simulink model "Assignment5"  (R2014a)
settings: Solver=FixedStepDiscrete  StartTime=0.0  StopTime=10.0  FixedStep=1  RelTol=1e-3
libraries: hdlsllib x19, simulink x6
settings Model: Creator=ramirezlara.h  LastModifiedBy=vu.du

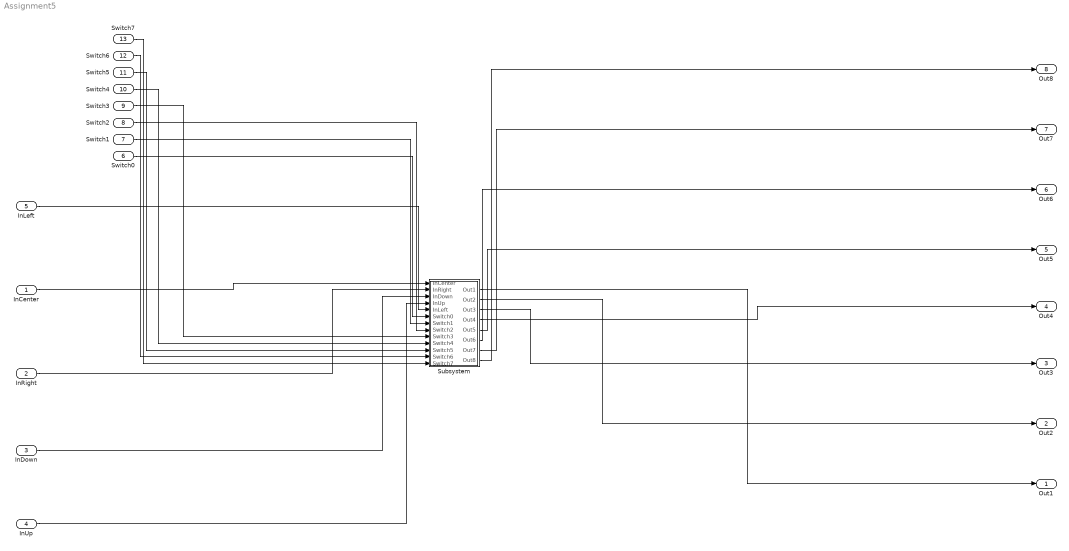
== system Assignment5 ==
  InCenter : Inport
  InRight : Inport  Port=2
  InDown : Inport  Port=3
  InUp : Inport  Port=4
  InLeft : Inport  Port=5
  Switch0 : Inport  Port=6  OutDataTypeStr=boolean
  Switch1 : Inport  Port=7  OutDataTypeStr=boolean
  Switch2 : Inport  Port=8  OutDataTypeStr=boolean
  Switch3 : Inport  Port=9  OutDataTypeStr=boolean
  Switch4 : Inport  Port=10  OutDataTypeStr=boolean
  Switch5 : Inport  Port=11  OutDataTypeStr=boolean
  Switch6 : Inport  Port=12  OutDataTypeStr=boolean
  Switch7 : Inport  Port=13  OutDataTypeStr=boolean
  Subsystem : Subsystem  TreatAsAtomicUnit=on
  Out1 : Outport
  Out2 : Outport  Port=2
  Out3 : Outport  Port=3
  Out4 : Outport  Port=4
  Out5 : Outport  Port=5
  Out6 : Outport  Port=6
  Out7 : Outport  Port=7
  Out8 : Outport  Port=8
  wires:
  InCenter/1 -> Subsystem/1(InCenter)
  InRight/1 -> Subsystem/2(InRight)
  InDown/1 -> Subsystem/3(InDown)
  InUp/1 -> Subsystem/4(InUp)
  InLeft/1 -> Subsystem/5(InLeft)
  Switch0/1 -> Subsystem/6(Switch0)
  Switch1/1 -> Subsystem/7(Switch1)
  Switch2/1 -> Subsystem/8(Switch2)
  Switch3/1 -> Subsystem/9(Switch3)
  Switch4/1 -> Subsystem/10(Switch4)
  Switch5/1 -> Subsystem/11(Switch5)
  Switch6/1 -> Subsystem/12(Switch6)
  Switch7/1 -> Subsystem/13(Switch7)
  Subsystem/1(Out1) -> Out1/1
  Subsystem/2(Out2) -> Out2/1
  Subsystem/3(Out3) -> Out3/1
  Subsystem/4(Out4) -> Out4/1
  Subsystem/5(Out5) -> Out5/1
  Subsystem/6(Out6) -> Out6/1
  Subsystem/7(Out7) -> Out7/1
  Subsystem/8(Out8) -> Out8/1

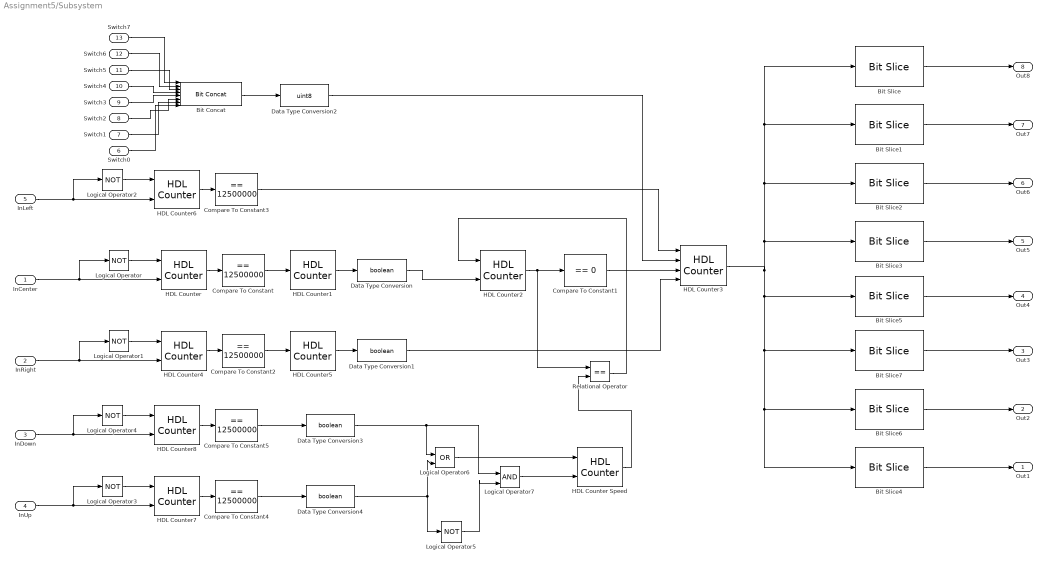
== system Assignment5/Subsystem ==
  InCenter : Inport
  InRight : Inport  Port=2
  InDown : Inport  Port=3
  InUp : Inport  Port=4
  InLeft : Inport  Port=5
  Switch0 : Inport  Port=6  OutDataTypeStr=boolean
  Switch1 : Inport  Port=7  OutDataTypeStr=boolean
  Switch2 : Inport  Port=8  OutDataTypeStr=boolean
  Switch3 : Inport  Port=9  OutDataTypeStr=boolean
  Switch4 : Inport  Port=10  OutDataTypeStr=boolean
  Switch5 : Inport  Port=11  OutDataTypeStr=boolean
  Switch6 : Inport  Port=12  OutDataTypeStr=boolean
  Switch7 : Inport  Port=13  OutDataTypeStr=boolean
  Bit Concat : hdlsllib/HDL Operations/Bit Concat  numInputs=8
  Bit Slice : hdlsllib/HDL Operations/Bit Slice  lidx=7  ridx=7
  Bit Slice1 : hdlsllib/HDL Operations/Bit Slice  lidx=6  ridx=6
  Bit Slice2 : hdlsllib/HDL Operations/Bit Slice  lidx=5  ridx=5
  Bit Slice3 : hdlsllib/HDL Operations/Bit Slice  lidx=4  ridx=4
  Bit Slice4 : hdlsllib/HDL Operations/Bit Slice  lidx=0  ridx=0
  Bit Slice5 : hdlsllib/HDL Operations/Bit Slice  lidx=3  ridx=3
  Bit Slice6 : hdlsllib/HDL Operations/Bit Slice  lidx=1  ridx=1
  Bit Slice7 : hdlsllib/HDL Operations/Bit Slice  lidx=2  ridx=2
  Compare To Constant{,2..5} (5 alike) : simulink/Logic and Bit Operations/Compare To Constant  relop===  const=12500000  OutDataTypeStr=boolean
  Compare To Constant1 : simulink/Logic and Bit Operations/Compare To Constant  relop===  const=0  OutDataTypeStr=boolean
  Data Type Conversion{,1,3..4} (4 alike) : DataTypeConversion  OutDataTypeStr=boolean
  Data Type Conversion2 : DataTypeConversion  OutDataTypeStr=uint8
  HDL Counter{,4,6..8} (5 alike) : hdlsllib/HDL Operations/HDL Counter  CountType=Count limited  CountInit=0  CountStep=1  CountMax=50000000  CountFromType=Initial value  CountFrom=0  CountResetPort=on  CountLoadPort=off  CountEnbPort=on  CountDirPort=off  CountDataType=Unsigned  CountWordLen=32  CountFracLen=0  CountSampTime=1
  HDL Counter Speed : hdlsllib/HDL Operations/HDL Counter  CountType=Free running  CountInit=25000000  CountStep=1000000  CountMax=50000000  CountFromType=Initial value  CountFrom=25000000  CountResetPort=off  CountLoadPort=off  CountEnbPort=on  CountDirPort=on  CountDataType=Unsigned  CountWordLen=32  CountFracLen=0  CountSampTime=1
  HDL Counter1 : hdlsllib/HDL Operations/HDL Counter  CountType=Free running  CountInit=0  CountStep=1  CountMax=100  CountFromType=Initial value  CountFrom=0  CountResetPort=off  CountLoadPort=off  CountEnbPort=on  CountDirPort=off  CountDataType=Unsigned  CountWordLen=1  CountFracLen=0  CountSampTime=1
  HDL Counter2 : hdlsllib/HDL Operations/HDL Counter  CountType=Free running  CountInit=0  CountStep=1  CountMax=25000000  CountFromType=Initial value  CountFrom=0  CountResetPort=on  CountLoadPort=off  CountEnbPort=on  CountDirPort=off  CountDataType=Unsigned  CountWordLen=32  CountFracLen=0  CountSampTime=1
  HDL Counter3 : hdlsllib/HDL Operations/HDL Counter  CountType=Free running  CountInit=0  CountStep=1  CountMax=25000000  CountFromType=Initial value  CountFrom=0  CountResetPort=off  CountLoadPort=on  CountEnbPort=on  CountDirPort=on  CountDataType=Unsigned  CountWordLen=8  CountFracLen=0  CountSampTime=1
  HDL Counter5 : hdlsllib/HDL Operations/HDL Counter  CountType=Free running  CountInit=1  CountStep=1  CountMax=100  CountFromType=Initial value  CountFrom=1  CountResetPort=off  CountLoadPort=off  CountEnbPort=on  CountDirPort=off  CountDataType=Unsigned  CountWordLen=1  CountFracLen=0  CountSampTime=1
  Logical Operator{,1..5} (6 alike) : Logic  Operator=NOT  IconShape=distinctive  AllPortsSameDT=off  OutDataTypeStr=boolean
  Logical Operator6 : Logic  Operator=OR  IconShape=distinctive  AllPortsSameDT=off  OutDataTypeStr=boolean
  Logical Operator7 : Logic  IconShape=distinctive  AllPortsSameDT=off  OutDataTypeStr=boolean
  Relational Operator : RelationalOperator  Operator===  OutDataTypeStr=boolean
  Out1 : Outport
  Out2 : Outport  Port=2
  Out3 : Outport  Port=3
  Out4 : Outport  Port=4
  Out5 : Outport  Port=5
  Out6 : Outport  Port=6
  Out7 : Outport  Port=7
  Out8 : Outport  Port=8
  wires:
  Data Type Conversion2/1 -> HDL Counter3/2
  Bit Slice3/1 -> Out5/1
  Data Type Conversion4/1 -> Logical Operator5/1, Logical Operator6/2
  Switch2/1 -> Bit Concat/6
  HDL Counter2/1 -> Relational Operator/1, Compare To Constant1/1
  Bit Slice4/1 -> Out1/1
  InUp/1 -> HDL Counter7/2, Logical Operator3/1
  Bit Concat/1 -> Data Type Conversion2/1
  Bit Slice5/1 -> Out4/1
  HDL Counter6/1 -> Compare To Constant3/1
  HDL Counter7/1 -> Compare To Constant4/1
  Bit Slice/1 -> Out8/1
  Switch6/1 -> Bit Concat/2
  Logical Operator4/1 -> HDL Counter8/1
  Bit Slice7/1 -> Out3/1
  InLeft/1 -> HDL Counter6/2, Logical Operator2/1
  Switch1/1 -> Bit Concat/7
  Switch7/1 -> Bit Concat/1
  HDL Counter1/1 -> Data Type Conversion/1
  Logical Operator3/1 -> HDL Counter7/1
  InCenter/1 -> HDL Counter/2, Logical Operator/1
  HDL Counter3/1 -> Bit Slice2/1, Bit Slice1/1, Bit Slice/1, Bit Slice3/1, Bit Slice6/1, Bit Slice4/1, Bit Slice7/1, Bit Slice5/1
  Logical Operator1/1 -> HDL Counter4/1
  InRight/1 -> HDL Counter4/2, Logical Operator1/1
  HDL Counter4/1 -> Compare To Constant2/1
  Logical Operator2/1 -> HDL Counter6/1
  HDL Counter5/1 -> Data Type Conversion1/1
  Compare To Constant1/1 -> HDL Counter3/3
  Logical Operator/1 -> HDL Counter/1
  Compare To Constant2/1 -> HDL Counter5/1
  Switch3/1 -> Bit Concat/5
  Data Type Conversion/1 -> HDL Counter2/2
  Data Type Conversion1/1 -> HDL Counter3/4
  Bit Slice1/1 -> Out7/1
  Compare To Constant3/1 -> HDL Counter3/1
  Switch0/1 -> Bit Concat/8
  Switch4/1 -> Bit Concat/4
  Bit Slice2/1 -> Out6/1
  Compare To Constant/1 -> HDL Counter1/1
  Switch5/1 -> Bit Concat/3
  HDL Counter/1 -> Compare To Constant/1
  HDL Counter8/1 -> Compare To Constant5/1
  Bit Slice6/1 -> Out2/1
  Compare To Constant5/1 -> Data Type Conversion3/1
  InDown/1 -> HDL Counter8/2, Logical Operator4/1
  Compare To Constant4/1 -> Data Type Conversion4/1
  Logical Operator6/1 -> HDL Counter Speed/1
  Logical Operator5/1 -> Logical Operator7/2
  Relational Operator/1 -> HDL Counter2/1
  HDL Counter Speed/1 -> Relational Operator/2
  Data Type Conversion3/1 -> Logical Operator7/1, Logical Operator6/1
  Logical Operator7/1 -> HDL Counter Speed/2
